simulink model "c10_wp_snake"  (R2021b)
settings: Solver=FixedStepDiscrete  StartTime=0.0  StopTime=Inf  FixedStep=sampleTime  RelTol=1e-3  EnableMultiTasking=on
InitFcn:
  | sampleTime = 0.05;
  | nMedianSize=3;
  | % Robot parameters
  | % Robot parameters
  | wheelRadius = 0.0303;
  | robotRadius = 0.116*0.8;   %小车在仿真中显示的圆形的半径大小
  | Trackwidth = 0.0847;  %定义向量场直方图算法中小车的宽度
  | 
  | % Lidar parameters
  | sensorOffset = [0,0];
  | scanAngles = linspace(-pi/3,pi/3,20)';%y = linspace(x1,x2,n) 生成 n 个点。这些点的间距为 (x2-x1)/(n-1)。
  | maxRange = 0.2;
  | 
  | %%%%%%
  | ks=1;
  | 
  | init_pose_1=[0    0  0]';
  | init_pose_2=[0    0.2  -pi/2]';
  | init_pose_3=[0    0.4  -pi/2]';
  | init_pose_4=[0    0.6  -pi/2]';
  | init_pose_5=[0    0.8  -pi/2]';
  | init_pose_6=[0    1  -pi/2]';
  | init_pose_7=[0    1.2  -pi/2]';
  | init_pose_8=[0    1.4  -pi/2]';
  | init_pose_9=[0    1.6  -pi/2]';
  | init_pose_10=[0   1.8  -pi/2]';
  | 
  | % paremeters of pure persuit
  | desired_v=0.2;
  | desired_w=2*pi;
  | desired_lookahead=0.2;
  | kv=0;
  | kw=1;%加速转弯
  | GoalRadius=0.15;%到达目标判定阈值
  | 
  | % paremeters of recovery
  | %recovery_w=0.5
  | recovery_w=2;
  | % Vector Field Histogram
  | numSector=180;%Number of angular sector
  | vehicleRadius=robotRadius;
  | rangeDis=[ 0, 0 ];%Range distance limits (m):
  | thresholds=[ 3, 8 ];%Histogram thresholds
  | %binary histogram 大于8是障碍物，小于3是空白区
  | %Thresholds for computing binary histogram, specified as a two-element vector of scalars. The algorithm uses these thresholds to compute the binary histogram from the polar obstacle density. Polar obstacle density values higher than the upper threshold are represented as occupied space (1) in the binary histogram. Values smaller than the lower threshold are represented as free space (0). Values that fall between the limits are set to the values of a previous computed binary histogram if one exists from previous iterations. If a previous histogram does not exist, the value is set as free space (0).
  | safetyDis=0.1;%Safety distance
  | minimumTurningRadius=0.5*robotRadius;%Minimum turning radius (m):
undefined symbols (not defined in the file): Angular, DiscIntNeverNeededParam, Linear
libraries: robotlib x42, dspstat3 x30, robotalgslib x20
(part 5 of 5)

== matlab function c10_wp_snake/Subsystem/Car Pose Listener9/Subsystem/sensor2vCar ==
  data: x_init output; y_init output; yaw_init output; flag output; poseNew input; poseMsg input
function [x_init,y_init,yaw_init,flag] = sensor2vCar(poseNew, poseMsg)
persistent x0 y0 yaw0 yaw1 x0_init y0_init yaw0_init fStart
if isempty(x0)
    x0=-10; y0=-10; yaw0=0; yaw1=0;   
    x0_init=-10;y0_init=-10;yaw0_init=0;
    fStart=0;
end
if poseNew
    if x0==poseMsg.Pose.Pose.Position.X&&y0==poseMsg.Pose.Pose.Position.Y
        flag=1;
    else
        x0=poseMsg.Pose.Pose.Position.X;
        y0=poseMsg.Pose.Pose.Position.Y;   
        %yaw2=atan2(2*(poseMsg.Pose.Pose.Orientation.Z*poseMsg.Pose.Pose.Orientation.W),1-2*(poseMsg.Pose.Pose.Orientation.Z^2)); 
        eul=quat2eul([poseMsg.Pose.Pose.Orientation.W,poseMsg.Pose.Pose.Orientation.X,poseMsg.Pose.Pose.Orientation.Y,poseMsg.Pose.Pose.Orientation.Z]);
        yaw2=eul(1);
        %对前后角度差使用积分，恢复yaw的连续性
        yaw0=yaw0+angdiff(yaw1,yaw2);
        yaw1=yaw2;
        flag=0;        
        x0_init=x0;
        y0_init=y0;
        yaw0_init=yaw0;
        fStart=1;
    end 
else
    if fStart
        flag=1;
    else
        flag=0;
    end
end

x_init=x0_init;y_init=y0_init;yaw_init=yaw0_init;

== matlab function c10_wp_snake/Subsystem/Car Pose Listener9/Subsystem/sensor2vCar4 ==
  data: V output; W output; VW_New input; VW_Msg input
function [V,W] = sensor2vCar(VW_New, VW_Msg)
persistent v0 w0
if isempty(v0)
    v0=0; 
    w0=0;    
end
if VW_New
    v0=VW_Msg.Linear.X;
    w0=VW_Msg.Angular.Z;
end

V=v0;
W=-w0;

== matlab function c10_wp_snake/controller/env/MATLAB Function9 ==
  data: poses input; idx input; ranges output; maxRange parameter; scanAngles parameter; robotRadius parameter

function ranges = genLidarSensor(poses,idx, maxRange, scanAngles, robotRadius)
%模拟激光雷达计算地图中障碍物距离

%计算部分
map=occupancyMap(3,3,50);
num=length(poses(1,:));%机器人总数
worldOffset=[0.5,0.5];%将世界坐标系偏移进地图
safetyDis=maxRange;
poseX=[poses(1,:)+worldOffset(1);poses(2,:)+worldOffset(2);poses(3,:)];
% for i=[1:idx-1 idx+1:num]
%     if poseX(i,1)>=0&&poseX(i,1)<=3&&poseX(i,2)>=0&&poseX(i,2)<=3        
%         setOccupancy(map,poseX(1:2,i)',1);
%     end
% end
obstacles = poseX(1:2,[1:idx-1 idx+1:num])';
setOccupancy(map,obstacles,ones(length(obstacles),1));
inflate(map,robotRadius);

if poseX(1,idx)>=0&&poseX(1,idx)<=3&&poseX(2,idx)>=0&&poseX(2,idx)<=3 
    vehiclePose = poseX(:,idx)';
    intsectionPts = rayIntersection(map,vehiclePose,scanAngles,safetyDis,0.7);
    offsets=intsectionPts-ones(length(scanAngles),1)*vehiclePose(1:2);
    ranges = sqrt(sum(offsets.^2,2));    
else
    ranges = nan(length(scanAngles),1);   
end

== matlab function c10_wp_snake/controller/Subsystem2/Compute Velocity and Heading for Path following/ Extract Goal ==
  data: Waypoints input; Goal output
function Goal = extractGoal(Waypoints)
%#codegen
b = isnan(Waypoints);
[rows,~] = find(b);
ridx = setdiff(1:size(Waypoints,1), sort(rows));
Goal = [Waypoints(ridx(end), 1) Waypoints(ridx(end), 2)];

== matlab function c10_wp_snake/controller/Subsystem3/Adjust Velocities to Avoid Obstacles/Path Following/Compute Angular Velocity ==
  data: steeringDir input; w output; wMax input
function w = exampleHelperComputeAngularVelocity(steeringDir, wMax)
%EXAMPLEHELPERCOMPUTEANGULARVELOCITY Compute angular velocity
%   W = exampleHelperComputeAngularVelocity(STEERINGDIR)
%   returns the angular velocity W for a differential drive robot in radians
%   per second for a given steering direction STEERINGDIR in the robot's
%   coordinate frame in radians.
%
%   W = exampleHelperComputeAngularVelocity(STEERINGDIR, WMAX)
%   returns the angular velocity W for a differential drive robot in radians
%   per second for a given steering direction STEERINGDIR in the robot's
%   coordinate frame in radians and maximum angular velocity WMAX in
%   radians per second. The output angular velocity is saturated based on
%   the WMAX.
%
%   Example:
%       
%       w = exampleHelperComputeAngularVelocity(0.2, 1);

% Copyright 2015 The MathWorks, Inc.

%#codegen
%#ok<*EMCA>

% Allow variable input arguments
if nargin == 1   
    wMax = inf;
end

validateattributes(steeringDir, {'double'},{'real'},...
    'exampleHelperComputeAngularVelocity', 'STEERINGDIR', 1);
validateattributes(wMax, {'double'},{'real', 'positive'},...
    'exampleHelperComputeAngularVelocity', 'WMAX', 2);

% Computing in robot's coordinate frame
curPose = [0 0 0];

% The following computation is similar to robotics.PurePursuit
lookaheadPoint = [cos(steeringDir), sin(steeringDir)];
slope = atan2((lookaheadPoint(2) - curPose(2)), ...
    (lookaheadPoint(1) - curPose(1)));
alpha = angdiff(curPose(3), slope);

% Angular velocity command for a differential drive robot is
% equal to the desired curvature to be followed by the robot.

w = (2*sin(alpha));

% Pick a constant rotation when robot is facing in the opposite
% direction of the path
if abs(abs(alpha) - pi) < 1e-12
    w = sign(w)*1;
end

if abs(w) > wMax
    w = sign(w)*wMax;
end

end

== matlab function c10_wp_snake/controller/Subsystem3/Compute Velocity and Heading for Path following/ Extract Goal ==
  data: Waypoints input; Goal output
function Goal = extractGoal(Waypoints)
%#codegen
b = isnan(Waypoints);
[rows,~] = find(b);
ridx = setdiff(1:size(Waypoints,1), sort(rows));
Goal = [Waypoints(ridx(end), 1) Waypoints(ridx(end), 2)];

== matlab function c10_wp_snake/controller/Subsystem4/Adjust Velocities to Avoid Obstacles/Path Following/Compute Angular Velocity ==
  data: steeringDir input; w output; wMax input
function w = exampleHelperComputeAngularVelocity(steeringDir, wMax)
%EXAMPLEHELPERCOMPUTEANGULARVELOCITY Compute angular velocity
%   W = exampleHelperComputeAngularVelocity(STEERINGDIR)
%   returns the angular velocity W for a differential drive robot in radians
%   per second for a given steering direction STEERINGDIR in the robot's
%   coordinate frame in radians.
%
%   W = exampleHelperComputeAngularVelocity(STEERINGDIR, WMAX)
%   returns the angular velocity W for a differential drive robot in radians
%   per second for a given steering direction STEERINGDIR in the robot's
%   coordinate frame in radians and maximum angular velocity WMAX in
%   radians per second. The output angular velocity is saturated based on
%   the WMAX.
%
%   Example:
%       
%       w = exampleHelperComputeAngularVelocity(0.2, 1);

% Copyright 2015 The MathWorks, Inc.

%#codegen
%#ok<*EMCA>

% Allow variable input arguments
if nargin == 1   
    wMax = inf;
end

validateattributes(steeringDir, {'double'},{'real'},...
    'exampleHelperComputeAngularVelocity', 'STEERINGDIR', 1);
validateattributes(wMax, {'double'},{'real', 'positive'},...
    'exampleHelperComputeAngularVelocity', 'WMAX', 2);

% Computing in robot's coordinate frame
curPose = [0 0 0];

% The following computation is similar to robotics.PurePursuit
lookaheadPoint = [cos(steeringDir), sin(steeringDir)];
slope = atan2((lookaheadPoint(2) - curPose(2)), ...
    (lookaheadPoint(1) - curPose(1)));
alpha = angdiff(curPose(3), slope);

% Angular velocity command for a differential drive robot is
% equal to the desired curvature to be followed by the robot.

w = (2*sin(alpha));

% Pick a constant rotation when robot is facing in the opposite
% direction of the path
if abs(abs(alpha) - pi) < 1e-12
    w = sign(w)*1;
end

if abs(w) > wMax
    w = sign(w)*wMax;
end

end

== matlab function c10_wp_snake/controller/Subsystem4/Compute Velocity and Heading for Path following/ Extract Goal ==
  data: Waypoints input; Goal output
function Goal = extractGoal(Waypoints)
%#codegen
b = isnan(Waypoints);
[rows,~] = find(b);
ridx = setdiff(1:size(Waypoints,1), sort(rows));
Goal = [Waypoints(ridx(end), 1) Waypoints(ridx(end), 2)];

== matlab function c10_wp_snake/controller/Subsystem5/Adjust Velocities to Avoid Obstacles/Path Following/Compute Angular Velocity ==
  data: steeringDir input; w output; wMax input
function w = exampleHelperComputeAngularVelocity(steeringDir, wMax)
%EXAMPLEHELPERCOMPUTEANGULARVELOCITY Compute angular velocity
%   W = exampleHelperComputeAngularVelocity(STEERINGDIR)
%   returns the angular velocity W for a differential drive robot in radians
%   per second for a given steering direction STEERINGDIR in the robot's
%   coordinate frame in radians.
%
%   W = exampleHelperComputeAngularVelocity(STEERINGDIR, WMAX)
%   returns the angular velocity W for a differential drive robot in radians
%   per second for a given steering direction STEERINGDIR in the robot's
%   coordinate frame in radians and maximum angular velocity WMAX in
%   radians per second. The output angular velocity is saturated based on
%   the WMAX.
%
%   Example:
%       
%       w = exampleHelperComputeAngularVelocity(0.2, 1);

% Copyright 2015 The MathWorks, Inc.

%#codegen
%#ok<*EMCA>

% Allow variable input arguments
if nargin == 1   
    wMax = inf;
end

validateattributes(steeringDir, {'double'},{'real'},...
    'exampleHelperComputeAngularVelocity', 'STEERINGDIR', 1);
validateattributes(wMax, {'double'},{'real', 'positive'},...
    'exampleHelperComputeAngularVelocity', 'WMAX', 2);

% Computing in robot's coordinate frame
curPose = [0 0 0];

% The following computation is similar to robotics.PurePursuit
lookaheadPoint = [cos(steeringDir), sin(steeringDir)];
slope = atan2((lookaheadPoint(2) - curPose(2)), ...
    (lookaheadPoint(1) - curPose(1)));
alpha = angdiff(curPose(3), slope);

% Angular velocity command for a differential drive robot is
% equal to the desired curvature to be followed by the robot.

w = (2*sin(alpha));

% Pick a constant rotation when robot is facing in the opposite
% direction of the path
if abs(abs(alpha) - pi) < 1e-12
    w = sign(w)*1;
end

if abs(w) > wMax
    w = sign(w)*wMax;
end

end

== matlab function c10_wp_snake/Subsystem/Car Pose Listener/Subsystem/sensor2vCar ==
  data: x_init output; y_init output; yaw_init output; flag output; poseNew input; poseMsg input
function [x_init,y_init,yaw_init,flag] = sensor2vCar(poseNew, poseMsg)
persistent x0 y0 yaw0 yaw1 x0_init y0_init yaw0_init fStart
if isempty(x0)
    x0=-10; y0=-10; yaw0=0; yaw1=0;   
    x0_init=-10;y0_init=-10;yaw0_init=0;
    fStart=0;
end
if poseNew
    if x0==poseMsg.Pose.Pose.Position.X&&y0==poseMsg.Pose.Pose.Position.Y
        flag=1;
    else
        x0=poseMsg.Pose.Pose.Position.X;
        y0=poseMsg.Pose.Pose.Position.Y;   
        %yaw2=atan2(2*(poseMsg.Pose.Pose.Orientation.Z*poseMsg.Pose.Pose.Orientation.W),1-2*(poseMsg.Pose.Pose.Orientation.Z^2)); 
        eul=quat2eul([poseMsg.Pose.Pose.Orientation.W,poseMsg.Pose.Pose.Orientation.X,poseMsg.Pose.Pose.Orientation.Y,poseMsg.Pose.Pose.Orientation.Z]);
        yaw2=eul(1);
        %对前后角度差使用积分，恢复yaw的连续性
        yaw0=yaw0+angdiff(yaw1,yaw2);
        yaw1=yaw2;
        flag=0;        
        x0_init=x0;
        y0_init=y0;
        yaw0_init=yaw0;
        fStart=1;
    end 
else
    if fStart
        flag=1;
    else
        flag=0;
    end
end

x_init=x0_init;y_init=y0_init;yaw_init=yaw0_init;
